simulink model "mcb_host_dsPIC33"  (R2020b)
settings: Solver=FixedStepDiscrete  StartTime=0.0  StopTime=inf  RelTol=1e-3  EnableMultiTasking=on
values from neighbouring files (symbols this model uses):
  Ts = T_pwm    (= 5e-05)    [mcb_pmsm_foc_sensorless_dsPIC33_data.m]
libraries: mcbhostblockslib x2, simulink x2
settings Model: Creator=The MathWorks, Inc.  LastModifiedBy=bmckay
settings DataIOCC: LimitDataPoints=on  SaveFormat=Array  ReturnWorkspaceOutputs=off
settings OptimizationCC: LifeSpan=1  EfficientTunableParamExpr=on
settings DebuggingCC: MergeDetectMultiDrivingBlocksExec=none  SolverPrmCheckMsg=warning  ParameterPrecisionLossMsg=none  AllowSymbolicDim=off  PregeneratedLibrarySubsystemCodeDiagnostic=none  SFUnexpectedBacktrackingDiag=warning  SFNoUnconditionalDefaultTransitionDiag=warning  SFExecutionAtInitializationDiag=none  ArithmeticOperatorsInVariantConditions=warning
settings HardwareCC: ProdBitPerPointer=32  ProdLargestAtomicFloat=None  ProdIntDivRoundTo=Undefined  ProdEndianess=Unspecified  ProdWordSize=32  ProdHWDeviceType=32-bit Generic
settings ModelReferenceCC: PropagateSignalLabelsOutOfModel=off
settings SFSimCC: SimUseLocalCustomCode=off  MATLABDynamicMemAlloc=off
settings RTWCC: Description=Real-Time Workshop Embedded Coder  SystemTargetFile=ert.tlc  TemplateMakefile=ert_default_tmf  GenerateReport=on  RTWUseLocalCustomCode=off  IncludeHyperlinkInReport=on  LaunchReport=on  GenerateTraceInfo=on  GenerateTraceReport=on  GenerateTraceReportSl=on  GenerateTraceReportSf=on  GenerateTraceReportEml=on
settings CodeAppCC: IgnoreCustomStorageClasses=off  StateflowObjectComments=on  InternalIdentifier=Classic
settings ERTTargetCC: MultiwordLength=2048  GenerateSampleERTMain=on  ERTCustomFileTemplate=example_file_process.tlc  ConvertIfToSwitch=off  SuppressUnreachableDefaultCases=off
settings ConfigComp: CovMetricSettings=dw  CovSaveCumulativeToWorkspaceVar=on  CovSaveSingleToWorkspaceVar=on  CovExternalEMLEnable=off  CovSFcnEnable=off

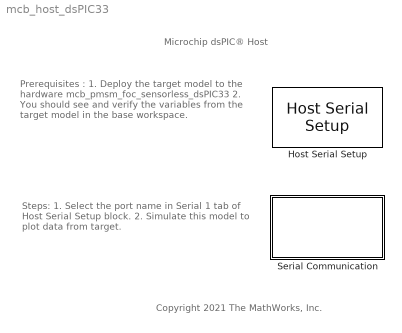
== system mcb_host_dsPIC33 ==
  note: Steps:
      | 1. Select the port name in Serial 1 tab of Host
      | Serial Setup block.
      | 2. Simulate this model to plot data from target.
  note: Prerequisites :
      | 1. Deploy the target model to the hardware
      | mcb_pmsm_foc_sensorless_dsPIC33
      | 2. You should see and verify the variables
      | from the target model in the base workspace.
  note: Microchip dsPIC® Host
  note: Copyright 2021 The MathWorks, Inc.
  Host Serial Setup : mcbhostblockslib/Host Serial Setup  Priority=-99  comPortSer1='COM5'  baudRateA=2916667  charLenA=8  stopBitA=1  parityA=none  timeoutA=2  ByteOrderA=LittleEndian  comPortSer2='Please_select_a_port'  baudRateB=115200  charLenB=8  stopBitB=1  parityB=none  timeoutB=1.0  ByteOrderB=LittleEndian  comPortSer3='Please_select_a_port'  baudRateC=115200  charLenC=8  stopBitC=1  parityC=none  timeoutC=1.0  ByteOrderC=LittleEndian  comPortSer4='Please_select_a_port'  baudRateD=115200  charLenD=8  stopBitD=1  parityD=none  timeoutD=1.0  ByteOrderD=LittleEndian
      settings: SourceProductBaseCode=MT
  Serial Communication : Subsystem

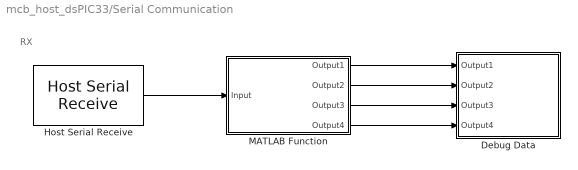
== system mcb_host_dsPIC33/Serial Communication ==
  note: RX
  Debug Data : Subsystem
  Host Serial Receive : mcbhostblockslib/Host Serial Receive  serialCon=Serial 1  dataHead='S'  dataTail='E'  dataType=uint8  dataDim=[600 4]  initValue=5  errOption=Output custom value  errValue=15  sampleTime=600 * Ts  outputStatus=off  blockingMode=on
      settings: SourceProductBaseCode=MT
  MATLAB Function : MATLAB Function  TreatAsAtomicUnit=on
  wires:
  Host Serial Receive/1 -> MATLAB Function/1(Input)
  MATLAB Function/1(Output1) -> Debug Data/1(Output1)
  MATLAB Function/2(Output2) -> Debug Data/2(Output2)
  MATLAB Function/3(Output3) -> Debug Data/3(Output3)
  MATLAB Function/4(Output4) -> Debug Data/4(Output4)

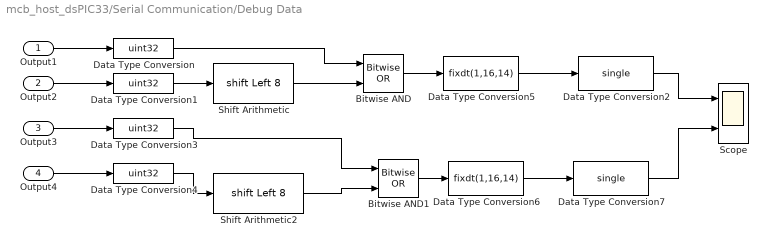
== system mcb_host_dsPIC33/Serial Communication/Debug Data ==
  Output1 : Inport
  Output2 : Inport  Port=2
  Output3 : Inport  Port=3
  Output4 : Inport  Port=4
  Bitwise AND : simulink/Logic and Bit Operations/Bitwise Operator  logicop=OR  UseBitMask=off  NumInputPorts=2  BitMask=bin2dec('11011001')  BitMaskRealWorld=Stored Integer
  Bitwise AND1 : simulink/Logic and Bit Operations/Bitwise Operator  logicop=OR  UseBitMask=off  NumInputPorts=2  BitMask=bin2dec('11011001')  BitMaskRealWorld=Stored Integer
  Data Type Conversion{,1,3..4} (4 alike) : DataTypeConversion  OutDataTypeStr=uint32  RndMeth=Simplest
  Data Type Conversion2 : DataTypeConversion  OutDataTypeStr=single  RndMeth=Simplest
  Data Type Conversion5 : DataTypeConversion  OutDataTypeStr=fixdt(1,16,14)  ConvertRealWorld=Stored Integer (SI)  RndMeth=Simplest
  Data Type Conversion6 : DataTypeConversion  OutDataTypeStr=fixdt(1,16,14)  ConvertRealWorld=Stored Integer (SI)  RndMeth=Simplest
  Data Type Conversion7 : DataTypeConversion  OutDataTypeStr=single  RndMeth=Simplest
  Scope : Scope  NumInputPorts=2
  Shift Arithmetic : ArithShift  BitShiftNumber=8  BitShiftDirection=Left
  Shift Arithmetic2 : ArithShift  BitShiftNumber=8  BitShiftDirection=Left
  wires:
  Output1/1 -> Data Type Conversion/1
  Data Type Conversion5/1 -> Data Type Conversion2/1
  Output2/1 -> Data Type Conversion1/1
  Bitwise AND/1 -> Data Type Conversion5/1
  Data Type Conversion1/1 -> Shift Arithmetic/1
  Data Type Conversion/1 -> Bitwise AND/1
  Data Type Conversion2/1 -> Scope/1
  Output3/1 -> Data Type Conversion3/1
  Output4/1 -> Data Type Conversion4/1
  Data Type Conversion4/1 -> Shift Arithmetic2/1
  Shift Arithmetic/1 -> Bitwise AND/2
  Bitwise AND1/1 -> Data Type Conversion6/1
  Data Type Conversion6/1 -> Data Type Conversion7/1
  Data Type Conversion7/1 -> Scope/2
  Data Type Conversion3/1 -> Bitwise AND1/1
  Shift Arithmetic2/1 -> Bitwise AND1/2

== matlab function mcb_host_dsPIC33/Serial Communication/MATLAB Function ==
  data: Output1 output; Output2 output; Input input; Output3 output; Output4 output
function [ Output1, Output2, Output3, Output4] = unBuf(Input)

Output1= Input(:, 1);
Output2 = Input(:, 2);
Output3 = Input(:, 3);
Output4 = Input(:, 4);
end
